simulink model "UAV"  (R2025b)
settings: Solver=ode3  StartTime=0.0  StopTime=inf  FixedStep=Sim.Ts_fisica  RelTol=1e-3
PostLoadFcn:
  | Init
InitFcn:
  | Init
model workspace (MAT data in the model file):
  Mass = 1
undefined symbols (not defined in the file): DiscIntNeverNeededParam, Drone, DWORK0, DWORK1, DWORK10, DWORK11, DWORK12, DWORK13, DWORK14, DWORK15, DWORK16, DWORK17, DWORK18, DWORK19, DWORK2, DWORK20, DWORK21, DWORK22, DWORK23, DWORK24, DWORK3, DWORK4, DWORK5, DWORK6, DWORK7, DWORK8, DWORK9, F, Light, MIL, Sim
libraries: simulink x35, slpidlib x11, vrlib x4, aerolibwind2 x2, sim3dlib x2, uavsim3dlib x2
(part 4 of 8)

== system UAV/untitledPanel3 ==
  Display1 : CustomWebBlock  Tag=HiddenForWebPanel  PanelInfo="{\"height\":50,\"left\":76,\"panelId\":\"panelId-c8b50f01-7e19-4994-ab96-2db03b8854f7\",\"top\":170,\"type\":\"panelChild\",\"version\":\"2019b\",\"width\":140,\"zIndex\":1500004}"  LabelPosition=Hide  ShowInitialText=on  Configuration="{\"components\":[{\"name\":\"DisplayComponent\",\"settings\":{\"bold\":true,\"font\":\"Roboto\",\"fontColor\":[255,255,255],\"fontSize\":\"23.621275710057528\",\"format\":\"Custom\",\"formatString\":\"%.1f m\",\"italic\":false,\"position\":[0,0.005194698952879581,0.9921875,1],\"underline\":false}},{\"name\":\"BackgroundImageComponent\",\"settings\":{\"image\":{\"size\":[140,50],\"src\":\"data:image\\/png;base64,iVBORw0KGgoAAAANSUhEUgAAAIwAAAAyCAIAAAABYqRsAAAACXBIWXMAAA7EAAAOxAGVKw4bAAAFU2lUWHRYTUw6Y29tLmFkb2JlLnhtcAAAAAAAPD94cGFja2V0IGJlZ2luPSfvu78nIGlkPSdXNU0wTXBDZWhpSHpyZVN6TlRjemtjOWQnPz4KPHg6eG1wbWV0YSB4bWxuczp4PSdhZG9iZTpuczptZXRhLyc+CjxyZGY6UkRGIHhtbG5zOnJkZj0naHR0cDovL3d3dy53My5vcmcvMTk5OS8wMi8yMi1yZGYtc3ludGF4LW5zIyc+CgogPHJkZjpEZXNjcmlwdGlvbiByZGY6YWJvdXQ9JycKICB4bWxuczpBdHRyaWI9J2h0dHA6Ly9ucy5h ...(+1856 chars)\",\"srcOrientation\":\"Right\"},\"position\":[0,0,1,1],\"scaleMode\":\"0\"}},{\"name\":\"ForegroundImageComponent\",\"settings\":{\"angle\":0,\"image\":{\"size\":[0,0],\"src\":\"default\"},\"isForeground\":1,\"position\":[0,0,1,1],\"scaleMode\":\"0\"}}],\"derived\":{\"blockParameters\":{\"fixedAspectRatio\":\"on\",\"format\":\"Custom\",\"formatString\":\"%.1f m\"}},\"settings\":{\"BindingType\":\"signal\",\"aspectRatio\":1.032258064516129,\"backgroundColor\":[0,0,0,\"1\"],\"backgroundOffset\":0.14,\"backgroundOpacity\":1,\"fixedAspectRatio\":\"on\",\"showBackgroundColor\":false,\"value\":0,\"version\":\"R2023b\"},\"type\":\"Display\"}"
  Display2 : CustomWebBlock  Tag=HiddenForWebPanel  PanelInfo="{\"height\":50,\"left\":78,\"panelId\":\"panelId-c8b50f01-7e19-4994-ab96-2db03b8854f7\",\"top\":269,\"type\":\"panelChild\",\"version\":\"2019b\",\"width\":140,\"zIndex\":1500026}"  LabelPosition=Hide  ShowInitialText=on  Configuration="{\"components\":[{\"name\":\"DisplayComponent\",\"settings\":{\"bold\":true,\"font\":\"Roboto\",\"fontColor\":[255,255,255],\"fontSize\":\"23.621275710057528\",\"format\":\"Custom\",\"formatString\":\"%.1f m\\/s\",\"italic\":false,\"position\":[0,0.005194698952879581,0.9921875,1],\"underline\":false}},{\"name\":\"BackgroundImageComponent\",\"settings\":{\"image\":{\"size\":[140,50],\"src\":\"data:image\\/png;base64,iVBORw0KGgoAAAANSUhEUgAAAIwAAAAyCAIAAAABYqRsAAAACXBIWXMAAA7EAAAOxAGVKw4bAAAFU2lUWHRYTUw6Y29tLmFkb2JlLnhtcAAAAAAAPD94cGFja2V0IGJlZ2luPSfvu78nIGlkPSdXNU0wTXBDZWhpSHpyZVN6TlRjemtjOWQnPz4KPHg6eG1wbWV0YSB4bWxuczp4PSdhZG9iZTpuczptZXRhLyc+CjxyZGY6UkRGIHhtbG5zOnJkZj0naHR0cDovL3d3dy53My5vcmcvMTk5OS8wMi8yMi1yZGYtc3ludGF4LW5zIyc+CgogPHJkZjpEZXNjcmlwdGlvbiByZGY6YWJvdXQ9JycKICB4bWxuczpBdHRyaWI9J2h0dHA6Ly9ucy5h ...(+1856 chars)\",\"srcOrientation\":\"Right\"},\"position\":[0,0,1,1],\"scaleMode\":\"0\"}},{\"name\":\"ForegroundImageComponent\",\"settings\":{\"angle\":0,\"image\":{\"size\":[0,0],\"src\":\"default\"},\"isForeground\":1,\"position\":[0,0,1,1],\"scaleMode\":\"0\"}}],\"derived\":{\"blockParameters\":{\"fixedAspectRatio\":\"on\",\"format\":\"Custom\",\"formatString\":\"%.1f m\\/s\"}},\"settings\":{\"BindingType\":\"signal\",\"aspectRatio\":1.032258064516129,\"backgroundColor\":[0,0,0,\"1\"],\"backgroundOffset\":0.14,\"backgroundOpacity\":1,\"fixedAspectRatio\":\"on\",\"showBackgroundColor\":false,\"value\":0,\"version\":\"R2023b\"},\"type\":\"Display\"}"
  Display3 : CustomWebBlock  Tag=HiddenForWebPanel  PanelInfo="{\"height\":45,\"left\":354,\"panelId\":\"panelId-c8b50f01-7e19-4994-ab96-2db03b8854f7\",\"top\":268,\"type\":\"panelChild\",\"version\":\"2019b\",\"width\":160,\"zIndex\":1500020}"  LabelPosition=Hide  ShowInitialText=on  Configuration="{\"components\":[{\"name\":\"DisplayComponent\",\"settings\":{\"bold\":true,\"font\":\"Roboto\",\"fontColor\":[255,255,255],\"fontSize\":\"23.621275710057528\",\"format\":\"Custom\",\"formatString\":\"%.0f s\",\"italic\":false,\"position\":[0,0.005194698952879581,0.9921875,1],\"underline\":false}},{\"name\":\"BackgroundImageComponent\",\"settings\":{\"image\":{\"size\":[160,45],\"src\":\"data:image\\/png;base64,iVBORw0KGgoAAAANSUhEUgAAAKAAAAAtCAIAAACmg\\/d8AAAACXBIWXMAAA7EAAAOxAGVKw4bAAAFRGlUWHRYTUw6Y29tLmFkb2JlLnhtcAAAAAAAPD94cGFja2V0IGJlZ2luPSfvu78nIGlkPSdXNU0wTXBDZWhpSHpyZVN6TlRjemtjOWQnPz4KPHg6eG1wbWV0YSB4bWxuczp4PSdhZG9iZTpuczptZXRhLyc+CjxyZGY6UkRGIHhtbG5zOnJkZj0naHR0cDovL3d3dy53My5vcmcvMTk5OS8wMi8yMi1yZGYtc3ludGF4LW5zIyc+CgogPHJkZjpEZXNjcmlwdGlvbiByZGY6YWJvdXQ9JycKICB4bWxuczpBdHRyaWI9J2h0dHA6Ly9ucy ...(+1822 chars)\",\"srcOrientation\":\"Right\"},\"position\":[0,0,1,1],\"scaleMode\":\"0\"}},{\"name\":\"ForegroundImageComponent\",\"settings\":{\"angle\":0,\"image\":{\"size\":[0,0],\"src\":\"default\"},\"isForeground\":1,\"position\":[0,0,1,1],\"scaleMode\":\"0\"}}],\"derived\":{\"blockParameters\":{\"fixedAspectRatio\":\"on\",\"format\":\"Custom\",\"formatString\":\"%.0f s\"}},\"settings\":{\"BindingType\":\"signal\",\"aspectRatio\":1.032258064516129,\"backgroundColor\":[0,0,0,\"1\"],\"backgroundOffset\":0.14,\"backgroundOpacity\":1,\"fixedAspectRatio\":\"on\",\"showBackgroundColor\":false,\"value\":0,\"version\":\"R2023b\"},\"type\":\"Display\"}"
  Display4 : CustomWebBlock  Tag=HiddenForWebPanel  PanelInfo="{\"height\":50,\"left\":74,\"panelId\":\"panelId-c8b50f01-7e19-4994-ab96-2db03b8854f7\",\"top\":71,\"type\":\"panelChild\",\"version\":\"2019b\",\"width\":140,\"zIndex\":1500002}"  LabelPosition=Hide  ShowInitialText=on  Configuration="{\"components\":[{\"name\":\"DisplayComponent\",\"settings\":{\"bold\":true,\"font\":\"Roboto\",\"fontColor\":[255,255,255],\"fontSize\":\"23.621275710057528\",\"format\":\"Custom\",\"formatString\":\"%.1f km\\/h\",\"italic\":false,\"position\":[0,0.005194698952879581,0.9921875,1],\"underline\":false}},{\"name\":\"BackgroundImageComponent\",\"settings\":{\"image\":{\"size\":[140,50],\"src\":\"data:image\\/png;base64,iVBORw0KGgoAAAANSUhEUgAAAIwAAAAyCAIAAAABYqRsAAAACXBIWXMAAA7EAAAOxAGVKw4bAAAFU2lUWHRYTUw6Y29tLmFkb2JlLnhtcAAAAAAAPD94cGFja2V0IGJlZ2luPSfvu78nIGlkPSdXNU0wTXBDZWhpSHpyZVN6TlRjemtjOWQnPz4KPHg6eG1wbWV0YSB4bWxuczp4PSdhZG9iZTpuczptZXRhLyc+CjxyZGY6UkRGIHhtbG5zOnJkZj0naHR0cDovL3d3dy53My5vcmcvMTk5OS8wMi8yMi1yZGYtc3ludGF4LW5zIyc+CgogPHJkZjpEZXNjcmlwdGlvbiByZGY6YWJvdXQ9JycKICB4bWxuczpBdHRyaWI9J2h0dHA6Ly9ucy5h ...(+1856 chars)\",\"srcOrientation\":\"Right\"},\"position\":[0,0,1,1],\"scaleMode\":\"0\"}},{\"name\":\"ForegroundImageComponent\",\"settings\":{\"angle\":0,\"image\":{\"size\":[0,0],\"src\":\"default\"},\"isForeground\":1,\"position\":[0,0,1,1],\"scaleMode\":\"0\"}}],\"derived\":{\"blockParameters\":{\"fixedAspectRatio\":\"on\",\"format\":\"Custom\",\"formatString\":\"%.1f km\\/h\"}},\"settings\":{\"BindingType\":\"signal\",\"aspectRatio\":1.032258064516129,\"backgroundColor\":[0,0,0,\"1\"],\"backgroundOffset\":0.14,\"backgroundOpacity\":1,\"fixedAspectRatio\":\"on\",\"showBackgroundColor\":false,\"value\":0,\"version\":\"R2023b\"},\"type\":\"Display\"}"
  Display5 : CustomWebBlock  Tag=HiddenForWebPanel  PanelInfo="{\"height\":39,\"left\":364,\"panelId\":\"panelId-c8b50f01-7e19-4994-ab96-2db03b8854f7\",\"top\":399,\"type\":\"panelChild\",\"version\":\"2019b\",\"width\":140,\"zIndex\":1500022}"  LabelPosition=Hide  ShowInitialText=on  Configuration="{\"components\":[{\"name\":\"DisplayComponent\",\"settings\":{\"bold\":true,\"font\":\"Roboto\",\"fontColor\":[255,255,255],\"fontSize\":\"23.621275710057528\",\"format\":\"Custom\",\"formatString\":\"%.1f %%\",\"italic\":false,\"position\":[0,0.005194698952879581,0.9921875,1],\"underline\":false}},{\"name\":\"BackgroundImageComponent\",\"settings\":{\"image\":{\"size\":[160,45],\"src\":\"data:image\\/png;base64,iVBORw0KGgoAAAANSUhEUgAAAKAAAAAtCAIAAACmg\\/d8AAAACXBIWXMAAA7EAAAOxAGVKw4bAAAFRGlUWHRYTUw6Y29tLmFkb2JlLnhtcAAAAAAAPD94cGFja2V0IGJlZ2luPSfvu78nIGlkPSdXNU0wTXBDZWhpSHpyZVN6TlRjemtjOWQnPz4KPHg6eG1wbWV0YSB4bWxuczp4PSdhZG9iZTpuczptZXRhLyc+CjxyZGY6UkRGIHhtbG5zOnJkZj0naHR0cDovL3d3dy53My5vcmcvMTk5OS8wMi8yMi1yZGYtc3ludGF4LW5zIyc+CgogPHJkZjpEZXNjcmlwdGlvbiByZGY6YWJvdXQ9JycKICB4bWxuczpBdHRyaWI9J2h0dHA6Ly9ucy ...(+1822 chars)\",\"srcOrientation\":\"Right\"},\"position\":[0,0,1,1],\"scaleMode\":\"0\"}},{\"name\":\"ForegroundImageComponent\",\"settings\":{\"angle\":0,\"image\":{\"size\":[0,0],\"src\":\"default\"},\"isForeground\":1,\"position\":[0,0,1,1],\"scaleMode\":\"0\"}}],\"derived\":{\"blockParameters\":{\"fixedAspectRatio\":\"on\",\"format\":\"Custom\",\"formatString\":\"%.1f %%\"}},\"settings\":{\"BindingType\":\"signal\",\"aspectRatio\":1.032258064516129,\"backgroundColor\":[0,0,0,\"1\"],\"backgroundOffset\":0.14,\"backgroundOpacity\":1,\"fixedAspectRatio\":\"on\",\"showBackgroundColor\":false,\"value\":0,\"version\":\"R2023b\"},\"type\":\"Display\"}"
  Heading Indicator : HeadingIndicatorBlock  Tag=HiddenForWebPanel  PanelInfo="{\"height\":200,\"left\":42,\"panelId\":\"panelId-c8b50f01-7e19-4994-ab96-2db03b8854f7\",\"top\":354,\"type\":\"panelChild\",\"version\":\"2019b\",\"width\":200,\"zIndex\":1500014}"  LabelPosition=Hide
  MultiStateImage1 : MultiStateImageBlock  Tag=HiddenForWebPanel  PanelInfo="{\"height\":45,\"left\":353,\"panelId\":\"panelId-c8b50f01-7e19-4994-ab96-2db03b8854f7\",\"top\":70,\"type\":\"panelChild\",\"version\":\"2019b\",\"width\":160,\"zIndex\":1500008}"  LabelPosition=Hide
  MultiStateImage2 : MultiStateImageBlock  Tag=HiddenForWebPanel  PanelInfo="{\"height\":45,\"left\":353,\"panelId\":\"panelId-c8b50f01-7e19-4994-ab96-2db03b8854f7\",\"top\":169,\"type\":\"panelChild\",\"version\":\"2019b\",\"width\":160,\"zIndex\":1500010}"  LabelPosition=Hide
  Vertical Gauge : CustomWebBlock  Tag=HiddenForWebPanel  PanelInfo="{\"height\":100,\"left\":346,\"panelId\":\"panelId-c8b50f01-7e19-4994-ab96-2db03b8854f7\",\"top\":438,\"type\":\"panelChild\",\"version\":\"2019b\",\"width\":180,\"zIndex\":1500024}"  LabelPosition=Hide  ShowInitialText=on  Configuration="{\"components\":[{\"name\":\"LinearScaleComponent\",\"settings\":{\"bounds\":{\"max\":100,\"min\":0,\"tickInterval\":\"auto\"},\"internalTickHeightScaleFactor\":1.6,\"labelColor\":[128,128,128],\"labelFont\":{\"font\":\"Arial\",\"fontSize\":12},\"labelOffset\":0.05,\"labelTransparency\":1,\"needleImage\":{\"size\":[0,0],\"src\":\"\"},\"needleOffset\":[0,0],\"needleSize\":{\"height\":0,\"width\":0},\"position\":[0.19205729166666666,0.08571428571428574,0.7442857142857143,0.6202799479166666],\"referencePoint\":\"auto\",\"scaleColors\":[],\"scaleColorsSize\":0.2,\"scaleDirection\":\"LR\",\"showLabels\":false,\"showMinorTicks\":0,\"showSpanLine\":false,\"showTicks\":false,\"tickColor\":[0,0,0],\"tickTransparency\":0.7,\"valueBarColor\":[230,230,230],\"valueBarOffset\":-0.09,\"valueBarSize\":0.96,\"valueBarTransparency\":1}},{\"name\":\"BackgroundImageComponent\",\"settings\":{\"image\":{\"size\":[232,418],\"src\":\"data:image\\/png;base64,iVBORw0KGgoAAAANSUhEUgAAAOgAAAGiCAYAAADtHYrGAAAAAXNSR0IArs4c6QAAAARnQU1BAACxjwv8YQUAAAAJcEhZcwAACxAAAAsQAa0jvXUAAAC0ZVhJZklJKgAIAAAABgASAQMAAQAAAAEAAAAaAQUAAQAAAFYAAAAbAQUAAQAAAF4AAAAoAQMAAQAAAAIAAAATAgMAAQAAAAEAAABphwQAAQAAAGYAAAAAAAAASAAAAAEAAABIAAAAAQAAAAYAAJAHAAQAAAAwMjEwAZEHAAQAAAABAgMAAKAHAAQAAAAwMTAwAaADAAEAAAD\\/\\/wAAAqAEAAEAAAAAAgAAA6AEAAEAAAAAAgAAAAAAAJFf8doAAAGHaVRYdFhNTDpjb20uYWRvYmUu ...(+3414 chars)\",\"srcOrientation\":\"Up\"},\"position\":[0,0,1,1],\"scaleMode\":\"0\"}},{\"name\":\"ForegroundImageComponent\",\"settings\":{\"image\":{\"size\":[0,0],\"src\":\"default\",\"srcOrientation\":[]},\"isForeground\":1,\"position\":[0,0,1,1],\"scaleMode\":\"0\"}}],\"derived\":{\"blockParameters\":{\"ForegroundColor\":[0,0,0],\"Limits\":{\"Max\":100,\"Min\":0,\"Ticks\":\"auto\"},\"ScaleColors\":[],\"ScaleDirection\":\"Clockwise\",\"ScaleMax\":100,\"ScaleMin\":0,\"TickInterval\":\"auto\",\"fixedAspectRatio\":\"on\"}},\"settings\":{\"BindingType\":\"signal\",\"backgroundColor\":[0,0,0,\"1\"],\"backgroundOffset\":0,\"backgroundOpacity\":1,\"fixedAspectRatio\":\"on\",\"orientation\":\"horizontal\",\"showBackgroundColor\":false,\"value\":0,\"version\":\"R2023a\"},\"type\":\"LinearGauge\"}"  CustomBackgroundColor="{\"color\":[0.8,0.8,0.8],\"show\":false}"
  panelInfo : PanelWebBlock  Tag=HiddenForWebPanel  PanelInfo="{\"compacted\":false,\"height\":596,\"isActiveTab\":true,\"left\":848,\"name\":\"Telemetry\",\"panelId\":\"panelId-c8b50f01-7e19-4994-ab96-2db03b8854f7\",\"popoutData\":{\"height\":691,\"left\":-1065,\"maximized\":false,\"top\":-333,\"width\":588},\"popoutMode\":\"window\",\"tabIndex\":0,\"tabbedSetId\":\"tabbedSet8974436027\",\"top\":86,\"type\":\"panel\",\"version\":\"2019b\",\"visible\":true,\"width\":576,\"zIndex\":1500008}"  PanelSnapshot=<binary blob, 71644 chars, not shown>  PanelBackground=data:image/png;base64,iVBORw0KGgoAAAANSUhEUgAAAkQAAAJYCAIAAAAMlm7tAAAAtGVYSWZJSSoACAAAAAYAEgEDAAEAAAABAAAAGgEFAAEAAABWAAAAGwEFAAEAAABeAAAAKAEDAAEAAAACAAAAEwIDAAEAAAABAAAAaYcEAAEAAABmAAAAAAAAAGAAAAABAAAAYAAAAAEAAAAGAACQBwAEAAAAMDIxMAGRBwAEAAAAAQIDAACgBwAEAAAAMDEwMAGgAwABAAAA//8AAAKgBAABAAAARAIAAAOgBAABAAAAWAIAAAAAAAD+dhaxAAAACXBIWXMAAA7EAAAOxAGVKw4bAAAFOmlUWHRYTUw6Y29tLmFkb2JlLnhtcAAAAAAAPD94cGFja2V0IGJlZ2luPSfvu78nIGlk ...(+14936 chars)

== system UAV/Flight Controller Software/Flight Controller Software MIL ==
  Pilot Inputs : Inport
  Power_Status : Inport  Port=2
  Measurements_In : Inport  Port=3
  Bus Creator : BusCreator  Inputs=4
  Bus Creator1 : BusCreator  Inputs=4
  Bus Creator2 : BusCreator  Inputs=4
  Bus Creator3 : BusCreator  Inputs=6
  Bus Creator4 : BusCreator  Inputs=6
  Bus Creator5 : BusCreator  Inputs=3
  Control Loops : Subsystem
  Flight Supervisor : Subsystem
  Mix Quad-X : Subsystem
  State Estimator : Subsystem
  Telemetry : Subsystem
  "Telemetry " : Outport
  PWM_Out : Outport  Port=2
  FR : Outport  Port=3
  wires:
  Control Loops/1(Fz) -> Bus Creator1/1, Mix Quad-X/1(Fz)
  Control Loops/2(T_Phi) -> Bus Creator1/2, Mix Quad-X/2(T_Phi)
  Control Loops/3(T_Psi) -> Bus Creator1/3, Mix Quad-X/3(T_Psi)
  Control Loops/4(T_Theta) -> Bus Creator1/4, Mix Quad-X/4(T_Theta)
  Measurements_In/1 -> State Estimator/2(" ")
  Bus Creator/1 -> PWM_Out/1
  Mix Quad-X/4(Motor 4) -> Bus Creator/4, Bus Creator2/4  "PWM_4"
  Mix Quad-X/3(Motor 3) -> Bus Creator/3, Bus Creator2/3  "PWM_3"
  Mix Quad-X/2(Motor 2) -> Bus Creator/2, Bus Creator2/2  "PWM_2"
  Mix Quad-X/1(Motor 1) -> Bus Creator/1, Bus Creator2/1  "PWM_1"
  Pilot Inputs/1 -> Flight Supervisor/1(Pilot Inputs)
  Power_Status/1 -> Flight Supervisor/2(Power_Status)
  Flight Supervisor/2(System Status) -> State Estimator/1(" System_Ready"), Bus Creator4/5, Control Loops/2(System Status), Bus Creator3/5  "System Status"
  State Estimator/1(Rates) -> Bus Creator4/4, Control Loops/3(Rates)  "Rates"
  State Estimator/2(Angles) -> Bus Creator4/3, Control Loops/4(Angles), Bus Creator3/3  "Angles"
  State Estimator/3(Pos) -> Bus Creator4/2, Control Loops/5(Pos), Bus Creator3/2  "Pos"
  State Estimator/4(Vel) -> Bus Creator4/1, Control Loops/6(Vel), Bus Creator3/1  "Vel"
  Flight Supervisor/1(Setpoints) -> Bus Creator4/6, Control Loops/1(Setpoints)  "Setpoints"
  Bus Creator3/1 -> Telemetry/1(Nav_Data)
  Telemetry/1("Tel_Out ") -> "Telemetry "/1
  Bus Creator5/1 -> FR/1
  Bus Creator2/1 -> Bus Creator5/1  "PWM_Motors"
  Bus Creator1/1 -> Bus Creator5/2  "Pid_Effort"
  Bus Creator4/1 -> Bus Creator5/3  "Nav_Data"
  State Estimator/5(DCMbe) -> Control Loops/7(DCMbe1)
